simulink library "constX_YZvarT_CNAPSTurb"  (R2018b)
settings: Solver=VariableStepAuto  StartTime=0.0  StopTime=10.0  RelTol=1e-3
undefined symbols (not defined in the file or in its folder): env
libraries: dspmtrx3 x5, Dynamic_2D_Lookup_Table x3
settings Model: Creator=jcreed2  LastModifiedBy=mcobb

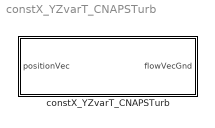
== system constX_YZvarT_CNAPSTurb ==
  constX_YZvarT_CNAPSTurb : Subsystem

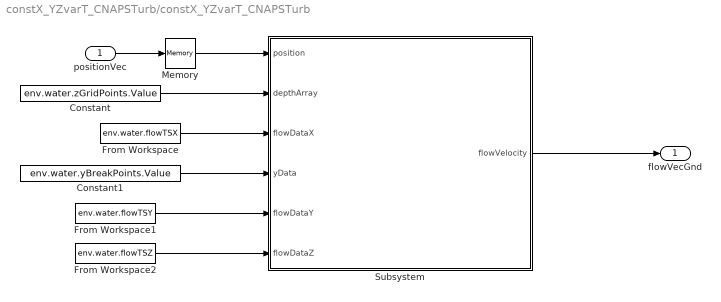
== system constX_YZvarT_CNAPSTurb/constX_YZvarT_CNAPSTurb ==
  "positionVec " : Inport
  Constant : Constant  Value=env.water.zGridPoints.Value
  Constant1 : Constant  Value=env.water.yBreakPoints.Value
  From Workspace : FromWorkspace  VariableName=env.water.flowTSX  SampleTime=0
  From Workspace1 : FromWorkspace  VariableName=env.water.flowTSY  SampleTime=0
  From Workspace2 : FromWorkspace  VariableName=env.water.flowTSZ  SampleTime=0
  Memory : Memory
  Subsystem : Subsystem
  flowVecGnd : Outport
  wires:
  From Workspace1/1 -> Subsystem/5("flowDataY ")
  "positionVec "/1 -> Memory/1
  Constant1/1 -> Subsystem/4("yData ")
  Subsystem/1("flowVelocity ") -> flowVecGnd/1
  From Workspace/1 -> Subsystem/3("flowDataX ")
  Constant/1 -> Subsystem/2("depthArray ")
  From Workspace2/1 -> Subsystem/6(flowDataZ)
  Memory/1 -> Subsystem/1("position ")

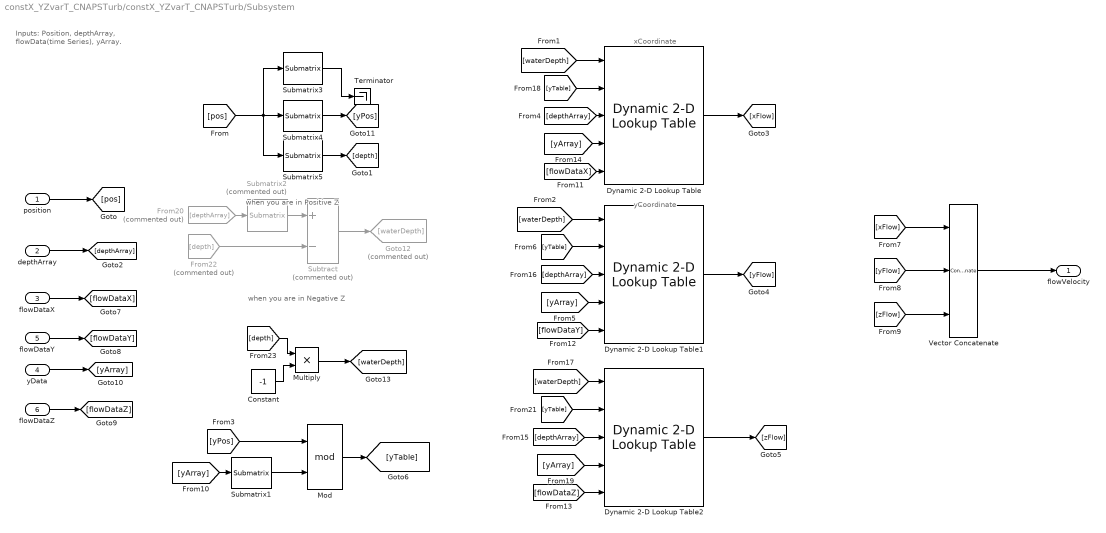
== system constX_YZvarT_CNAPSTurb/constX_YZvarT_CNAPSTurb/Subsystem ==
  note: when you are in Negative Z
  note: when you are in Positive Z
  note: yCoordinate
  note: xCoordinate
  note: Inputs: Position, depthArray,
      | flowData(time Series), yArray.
  "position " : Inport
  "depthArray " : Inport  Port=2
  "flowDataX " : Inport  Port=3
  "yData " : Inport  Port=4
  "flowDataY " : Inport  Port=5
  flowDataZ : Inport  Port=6
  Constant : Constant  Value=-1
  Dynamic 2-D Lookup Table : Dynamic_2D_Lookup_Table/Dynamic 2-D Lookup Table
  Dynamic 2-D Lookup Table1 : Dynamic_2D_Lookup_Table/Dynamic 2-D Lookup Table
  Dynamic 2-D Lookup Table2 : Dynamic_2D_Lookup_Table/Dynamic 2-D Lookup Table
  From20 : From  Commented=on  GotoTag=depthArray
  From22 : From  Commented=on  GotoTag=depth
  Goto12 : Goto  Commented=on  GotoTag=waterDepth
  Mod : Math  Operator=mod  SaturateOnIntegerOverflow=on
  Multiply : Product
  Submatrix1 : dspmtrx3/Submatrix  RowSpan=One row  RowStartMode=Last  RowStartIndex=1  RowEndMode=Last  RowEndIndex=1  ColSpan=All columns  ColStartMode=Last  ColStartIndex=1  ColEndMode=Last  ColEndIndex=1
  Submatrix2 : dspmtrx3/Submatrix  Commented=on  RowSpan=One row  RowStartMode=Last  RowStartIndex=1  RowEndMode=Last  RowEndIndex=1  ColSpan=All columns  ColStartMode=Last  ColStartIndex=1  ColEndMode=Last  ColEndIndex=1
  Submatrix3 : dspmtrx3/Submatrix  RowSpan=One row  RowStartMode=First  RowStartIndex=1  RowEndMode=Last  RowEndIndex=1  ColSpan=All columns  ColStartMode=First  ColStartIndex=1  ColEndMode=Last  ColEndIndex=1
  Submatrix4 : dspmtrx3/Submatrix  RowSpan=One row  RowStartMode=Middle  RowStartIndex=1  RowEndMode=Last  RowEndIndex=1  ColSpan=All columns  ColStartMode=First  ColStartIndex=1  ColEndMode=Last  ColEndIndex=1
  Submatrix5 : dspmtrx3/Submatrix  RowSpan=One row  RowStartMode=Last  RowStartIndex=1  RowEndMode=Last  RowEndIndex=1  ColSpan=All columns  ColStartMode=First  ColStartIndex=1  ColEndMode=Last  ColEndIndex=1
  Subtract : Sum  Commented=on  Inputs=+-
  Terminator : Terminator
  Vector Concatenate : Concatenate  NumInputs=3  Mode=Multidimensional array
  "flowVelocity " : Outport
  wires:
  [yPos] -> Mod/1
  [yTable] -> Dynamic 2-D Lookup Table1/2
  "position "/1 -> [pos]
  [depthArray] -> Dynamic 2-D Lookup Table/3
  [yArray] -> Submatrix1/1
  Submatrix5/1 -> [depth]
  [waterDepth] -> Dynamic 2-D Lookup Table1/1
  [depthArray] -> Dynamic 2-D Lookup Table1/3
  Submatrix3/1 -> Terminator/1
  [xFlow] -> Vector Concatenate/1
  Subtract/1 -> Goto12/1
  [flowDataY] -> Dynamic 2-D Lookup Table1/5
  Mod/1 -> [yTable]
  From22/1 -> Subtract/2
  [waterDepth] -> Dynamic 2-D Lookup Table/1
  [yFlow] -> Vector Concatenate/2
  [pos] -> Submatrix4/1, Submatrix5/1, Submatrix3/1
  "depthArray "/1 -> [depthArray]
  "flowDataY "/1 -> [flowDataY]
  Submatrix4/1 -> [yPos]
  Dynamic 2-D Lookup Table/1 -> [xFlow]
  Vector Concatenate/1 -> "flowVelocity "/1
  "yData "/1 -> [yArray]
  Submatrix1/1 -> Mod/2
  Dynamic 2-D Lookup Table1/1 -> [yFlow]
  [flowDataX] -> Dynamic 2-D Lookup Table/5
  [yArray] -> Dynamic 2-D Lookup Table1/4
  [yArray] -> Dynamic 2-D Lookup Table/4
  From20/1 -> Submatrix2/1
  [zFlow] -> Vector Concatenate/3
  "flowDataX "/1 -> [flowDataX]
  [yTable] -> Dynamic 2-D Lookup Table/2
  Submatrix2/1 -> Subtract/1
  Dynamic 2-D Lookup Table2/1 -> [zFlow]
  [waterDepth] -> Dynamic 2-D Lookup Table2/1
  [yArray] -> Dynamic 2-D Lookup Table2/4
  [depthArray] -> Dynamic 2-D Lookup Table2/3
  [yTable] -> Dynamic 2-D Lookup Table2/2
  flowDataZ/1 -> [flowDataZ]
  [flowDataZ] -> Dynamic 2-D Lookup Table2/5
  [depth] -> Multiply/1
  Constant/1 -> Multiply/2
  Multiply/1 -> [waterDepth]
